simulink model "HVAC"  (R2018a)
settings: Solver=VariableStepAuto  StartTime=0.0  StopTime=10.0  RelTol=1e-3
libraries: arduinolib x6
settings Model: Creator=yupuic  LastModifiedBy=yupuic
settings DataIOCC: ExternalInput=[t, in1],[t, in2],[t, in3]  LoadExternalInput=on

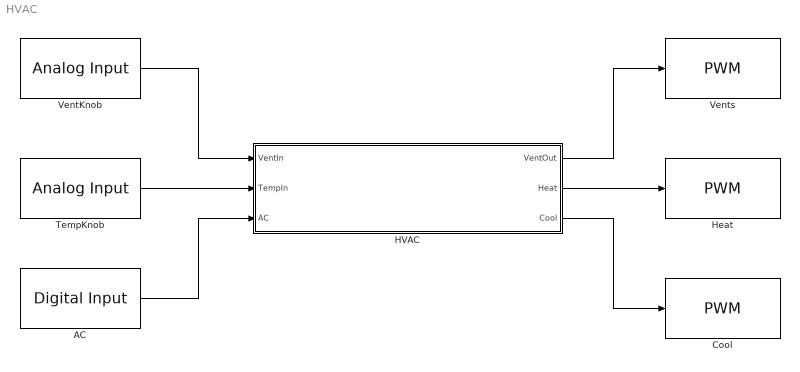
== system HVAC ==
  "AC " : arduinolib/Digital Input  pinNumber=7  sampleTime=0.1  blockPlatform=arduino
      settings: SourceProductName=Simulink Support Package for Arduino Hardware
  Cool : arduinolib/PWM  pinNumber=11  EnableInputFrequency=off  InitialFrequency=2000  InitialDutyCycle=0  NotificationType=None  blockPlatform=arduino
  HVAC : Subsystem
  Heat : arduinolib/PWM  pinNumber=10  EnableInputFrequency=off  InitialFrequency=2000  InitialDutyCycle=0  NotificationType=None  blockPlatform=arduino
  TempKnob : arduinolib/Analog Input  pinNumber=1  ReadResultsOnly=off  ConversionTriggerSource=Software  ExternalTriggerType=uint32(0)  OutputDataType=uint16  EnableConversionCompleteNotify=off  EnableOuputStatus=off  SampleTime=1  blockPlatform=arduino
  VentKnob : arduinolib/Analog Input  pinNumber=0  ReadResultsOnly=off  ConversionTriggerSource=Software  ExternalTriggerType=uint32(0)  OutputDataType=uint16  EnableConversionCompleteNotify=off  EnableOuputStatus=off  SampleTime=1  blockPlatform=arduino
  "Vents " : arduinolib/PWM  pinNumber=9  EnableInputFrequency=off  InitialFrequency=2000  InitialDutyCycle=0  NotificationType=None  blockPlatform=arduino
  wires:
  TempKnob/1 -> HVAC/2(TempIn)
  VentKnob/1 -> HVAC/1(VentIn)
  "AC "/1 -> HVAC/3(AC)
  HVAC/2(Heat) -> Heat/1
  HVAC/1(VentOut) -> "Vents "/1
  HVAC/3(Cool) -> Cool/1

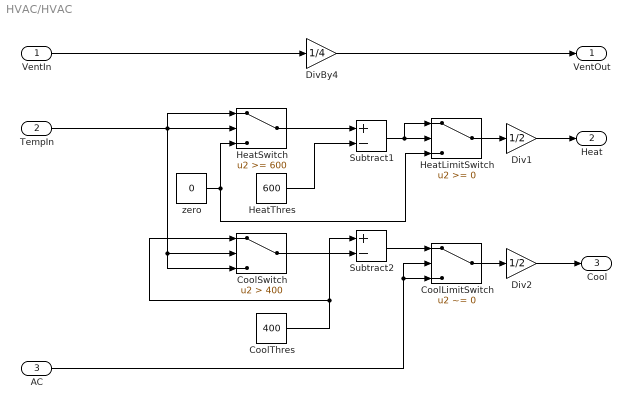
== system HVAC/HVAC ==
  VentIn : Inport
  TempIn : Inport  Port=2
  AC : Inport  Port=3
  CoolLimitSwitch : Switch  Criteria=u2 ~= 0
  CoolSwitch : Switch  Criteria=u2 > Threshold  Threshold=400
  CoolThres : Constant  Value=400
  Div1 : Gain  Gain=1/2
  Div2 : Gain  Gain=1/2
  DivBy4 : Gain  Gain=1/4
  HeatLimitSwitch : Switch
  HeatSwitch : Switch  Threshold=600
  HeatThres : Constant  Value=600
  Subtract1 : Sum  Inputs=+-
  Subtract2 : Sum  Inputs=+-
  zero : Constant  Value=0
  VentOut : Outport
  Heat : Outport  Port=2
  Cool : Outport  Port=3
  wires:
  CoolSwitch/1 -> Subtract2/2
  Div2/1 -> Cool/1
  VentIn/1 -> DivBy4/1
  zero/1 -> HeatSwitch/3, HeatLimitSwitch/3
  AC/1 -> CoolLimitSwitch/2, CoolLimitSwitch/3
  Subtract2/1 -> CoolLimitSwitch/1
  HeatSwitch/1 -> Subtract1/1
  CoolLimitSwitch/1 -> Div2/1
  HeatThres/1 -> Subtract1/2
  CoolThres/1 -> CoolSwitch/1, Subtract2/1
  TempIn/1 -> HeatSwitch/1, HeatSwitch/2, CoolSwitch/3, CoolSwitch/2
  Subtract1/1 -> HeatLimitSwitch/1, HeatLimitSwitch/2
  HeatLimitSwitch/1 -> Div1/1
  DivBy4/1 -> VentOut/1
  Div1/1 -> Heat/1
